simulink model "MBSE_drone_project_stateflow(1)"  (R2023a)
settings: Solver=FixedStepDiscrete  StartTime=0.0  StopTime=10.0  FixedStep=0.1  RelTol=1e-3  EnableMultiTasking=on
settings Model: Creator=tiesd  LastModifiedBy=tiesd
settings SolverCC: AlgebraicLoopSolver=TrustRegion  AutoInsertRateTranBlk=on
settings DataIOCC: LimitDataPoints=on
settings OptimizationCC: LifeSpan=inf
settings DebuggingCC: UnconnectedInputMsg=warning  UnconnectedOutputMsg=warning  UnconnectedLineMsg=warning  AllowSymbolicDim=off  SFUnexpectedBacktrackingDiag=warning  SFNoUnconditionalDefaultTransitionDiag=warning  SFExecutionAtInitializationDiag=none  ArithmeticOperatorsInVariantConditions=warning
settings ModelReferenceCC: EnableRefExpFcnMdlSchedulingChecks=on
settings SFSimCC: SimUseLocalCustomCode=off  CustomCodeUndefinedFunction=UseInterfaceOnly
settings RTWCC: RTWUseLocalCustomCode=off  DLArmComputeVersion=19.05
settings CodeAppCC: StateflowObjectComments=on
settings GRTTargetCC: TargetLangStandard=C89/C90 (ANSI)
settings ConfigComp: CovMetricSettings=dw  CovSaveCumulativeToWorkspaceVar=on  CovSaveSingleToWorkspaceVar=on  CovExternalEMLEnable=off  CovSFcnEnable=off

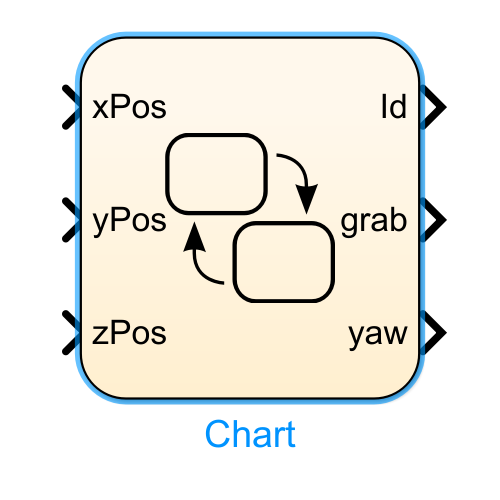
[thumbnail: Simulink's stored preview of the top-level diagram]
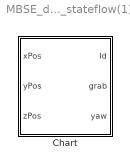
== system MBSE_drone_project_stateflow(1) ==
  Chart : Stateflow chart  TreatAsAtomicUnit=on

== stateflow chart MBSE_drone_project_stateflow(1)/Chart ==
  state Land
    entry:
    Id=1;
  state GoToDrop
    entry:
    x=2;
    y=0;
    z=-0.5;
    Id=0;
  state Drop
    entry:
    grab = 0;
  state Turn
    entry:
    x=2;
    y=0;
    z=-1.3;
    Id=0;
    yaw=3.1415;
  state LiftOff
    entry:
    x = 0;
    y = 0;
    z = -1;
    Id = 0;
    grab = 1;
    yaw = 0;
    delay = 2;
  state FindDrop
    entry:
    x = 0;
    y = 0;
    z = -1.3;
    Id = 0;
  state GoHome
    entry:
    x=0;
    y=0;
    z=-1;
    Id=0;
  (default) -> LiftOff
  Drop -> Turn : [((xPos <=x+0.1)&&(xPos>=x-0.1))&&((yPos<=y+0.1)&&(yPos>=y-0.1))&&((zPos<=z+0.1)&&(zPos>=z-0.1))&&after(delay,sec)]
  GoToDrop -> Drop : [((xPos <=x+0.1)&&(xPos>=x-0.1))&&((yPos<=y+0.1)&&(yPos>=y-0.1))&&((zPos<=z+0.1)&&(zPos>=z-0.1))&&after(delay,sec)]
  FindDrop -> GoToDrop : [((xPos <=x+0.1)&&(xPos>=x-0.1))&&((yPos<=y+0.1)&&(yPos>=y-0.1))&&((zPos<=z+0.1)&&(zPos>=z-0.1))&&after(delay,sec)]
  Turn -> GoHome : [((xPos <=x+0.1)&&(xPos>=x-0.1))&&((yPos<=y+0.1)&&(yPos>=y-0.1))&&((zPos<=z+0.1)&&(zPos>=z-0.1))&&after(delay,sec)]
  LiftOff -> FindDrop : [((xPos <=x+0.1)&&(xPos>=x-0.1))&&((yPos<=y+0.1)&&(yPos>=y-0.1))&&((zPos<=z+0.1)&&(zPos>=z-0.1))&&after(delay,sec)]
  GoHome -> Land : [((xPos <=x+0.1)&&(xPos>=x-0.1))&&((yPos<=y+0.1)&&(yPos>=y-0.1))&&((zPos<=z+0.1)&&(zPos>=z-0.1))&&after(delay,sec)]
  data: x local; xPos input; yPos input; zPos input; Id output; grab output; yaw output; delay local; y local; z local
